simulink model "fe_detect"  (R2018b)
settings: Solver=FixedStepAuto  StartTime=0.0  StopTime=10.0  FixedStep=1  RelTol=1e-3
libraries: simulink x2
settings Model: Creator=jason  LastModifiedBy=jason
settings OptimizationCC: DefaultParameterBehavior=Inlined

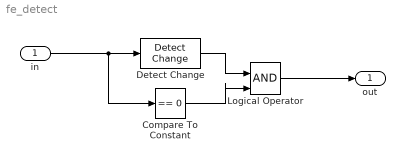
== system fe_detect ==
  in : Inport  OutDataTypeStr=boolean
  Compare To Constant : simulink/Logic and Bit Operations/Compare To Constant  relop===  const=0  OutDataTypeStr=boolean
  Detect Change : simulink/Logic and Bit Operations/Detect Change  vinit=0  OutDataTypeStr=boolean
  Logical Operator : Logic  IconShape=distinctive  AllPortsSameDT=off  OutDataTypeStr=boolean
  out : Outport  OutDataTypeStr=boolean
  wires:
  Detect Change/1 -> Logical Operator/1
  in/1 -> Compare To Constant/1, Detect Change/1
  Compare To Constant/1 -> Logical Operator/2
  Logical Operator/1 -> out/1
